simulink model "radarSim3"  (R2023b)
settings: Solver=VariableStepAuto  StartTime=0.0  StopTime=simTime  RelTol=1e-3
values from neighbouring files (symbols this model uses):
  c = get(groot,'defaultAxesColorOrder')    [compareData.m]
undefined symbols (not defined in the file or in its folder): fs, txDf_Dt, windowLen
libraries: dspsrcs4 x4, dspstat3 x2, dspxfrm3 x2
settings Model: Creator=pbroo  LastModifiedBy=pbroo

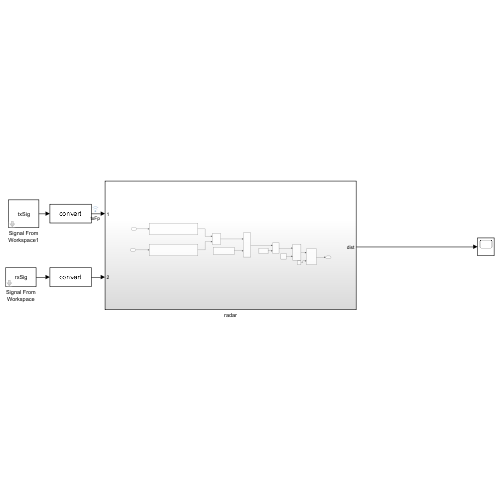
[thumbnail: Simulink's stored preview of the top-level diagram]
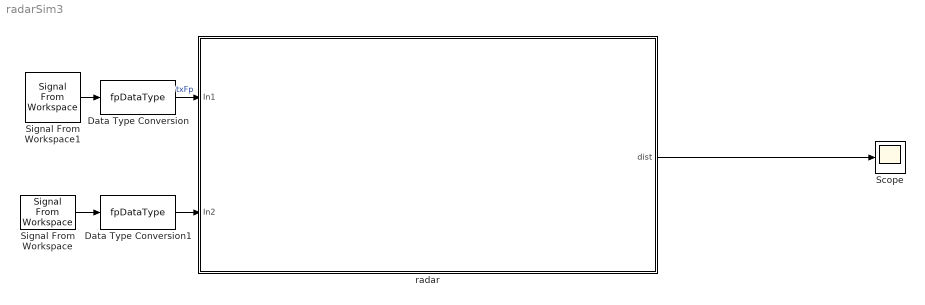
== system radarSim3 ==
  Data Type Conversion : DataTypeConversion  OutDataTypeStr=fpDataType  SaturateOnIntegerOverflow=off  RndMeth=Floor
  Data Type Conversion1 : DataTypeConversion  OutDataTypeStr=fpDataType  SaturateOnIntegerOverflow=off  RndMeth=Floor
  Scope : Scope
  Signal From Workspace : dspsrcs4/Signal From Workspace  X=rxSig  Ts=1  nsamps=1  OutputAfterFinalValue=Setting to zero  ignoreOrWarnInputAndFrameLengths=off  OutputFrames=off
  Signal From Workspace1 : dspsrcs4/Signal From Workspace  X=txSig  Ts=1  nsamps=1  OutputAfterFinalValue=Setting to zero  ignoreOrWarnInputAndFrameLengths=off  OutputFrames=off
  radar : Subsystem
  wires:
  Signal From Workspace1/1 -> Data Type Conversion/1
  Signal From Workspace/1 -> Data Type Conversion1/1
  radar/1(dist) -> Scope/1
  Data Type Conversion/1 -> radar/1(In1)  "txFp"
  Data Type Conversion1/1 -> radar/2(In2)

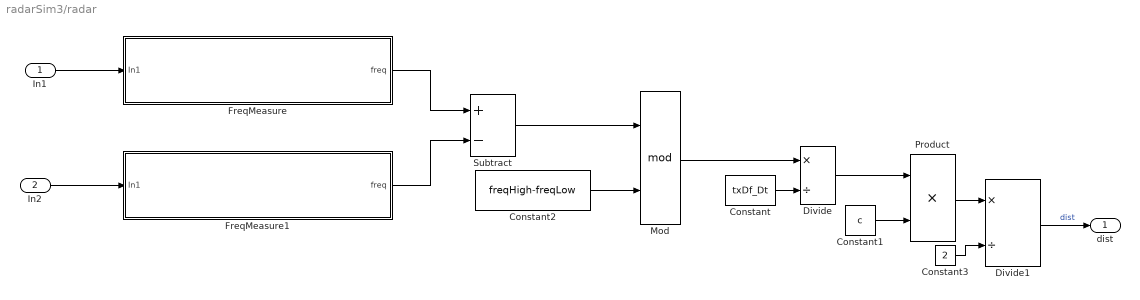
== system radarSim3/radar ==
  In1 : Inport
  In2 : Inport  Port=2
  Constant : Constant  Value=txDf_Dt
  Constant1 : Constant  Value=c
  Constant2 : Constant  Value=freqHigh-freqLow
  Constant3 : Constant  Value=2  VectorParams1D=off  SampleTime=-1
  Divide : Product  Inputs=*/
  Divide1 : Product  Inputs=*/
  FreqMeasure : Subsystem
  FreqMeasure1 : Subsystem
  Mod : Math  Operator=mod  SignedPower=on
  Product : Product
  Subtract : Sum  Inputs=+-
  dist : Outport
  wires:
  Subtract/1 -> Mod/1
  FreqMeasure1/1(freq) -> Subtract/2
  Constant/1 -> Divide/2
  Mod/1 -> Divide/1
  Divide/1 -> Product/1
  Constant1/1 -> Product/2
  FreqMeasure/1(freq) -> Subtract/1
  Constant2/1 -> Mod/2
  In1/1 -> FreqMeasure/1(In1)
  In2/1 -> FreqMeasure1/1(In1)
  Product/1 -> Divide1/1
  Divide1/1 -> dist/1  "dist"
  Constant3/1 -> Divide1/2

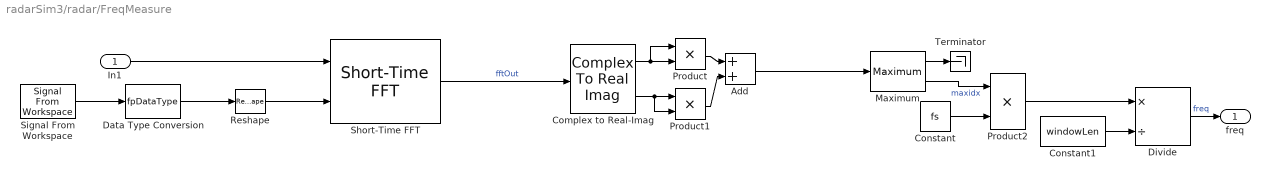
== system radarSim3/radar/FreqMeasure ==
  In1 : Inport
  Add : Sum
  Complex to Real-Imag : ComplexToRealImag
  Constant : Constant  Value=fs
  Constant1 : Constant  Value=windowLen
  Data Type Conversion : DataTypeConversion  OutDataTypeStr=fpDataType  SaturateOnIntegerOverflow=off  RndMeth=Floor
  Divide : Product  Inputs=*/
  Maximum : dspstat3/Maximum  operation=maximum  fcn=Value and Index  indexBase=One  operateOver=Each column  Dimension=1  InputProcessing=Columns as channels (frame based)  reset=None  roiEnable=off  roiType=Rectangles  roiPortion=Entire ROI  roiOutput=Individual statistics for each ROI  roiFlag=off  roundingMode=Floor  overflowMode=off  accumDataTypeStr=Inherit: Same as product output  accumLastDataTypeStr=Inherit: Same as product output
  Product : Product
  Product1 : Product
  Product2 : Product
  Reshape : Reshape  OutputDimensionality=Column vector (2-D)
  Short-Time FFT : dspxfrm3/Short-Time FFT  W=windowLen  OvLap=nOverlap  M=windowLen
  Signal From Workspace : dspsrcs4/Signal From Workspace  X=window  Ts=1  nsamps=1  OutputAfterFinalValue=Setting to zero  ignoreOrWarnInputAndFrameLengths=off  OutputFrames=off
  Terminator : Terminator
  freq : Outport
  wires:
  Maximum/2 -> Product2/1  "maxidx"
  Add/1 -> Maximum/1
  Constant1/1 -> Divide/2
  Constant/1 -> Product2/2
  Product2/1 -> Divide/1
  Divide/1 -> freq/1  "freq"
  Maximum/1 -> Terminator/1
  Short-Time FFT/1 -> Complex to Real-Imag/1  "fftOut"
  In1/1 -> Short-Time FFT/1
  Complex to Real-Imag/1 -> Product/1, Product/2
  Complex to Real-Imag/2 -> Product1/2, Product1/1
  Product/1 -> Add/1
  Product1/1 -> Add/2
  Signal From Workspace/1 -> Data Type Conversion/1
  Reshape/1 -> Short-Time FFT/2
  Data Type Conversion/1 -> Reshape/1

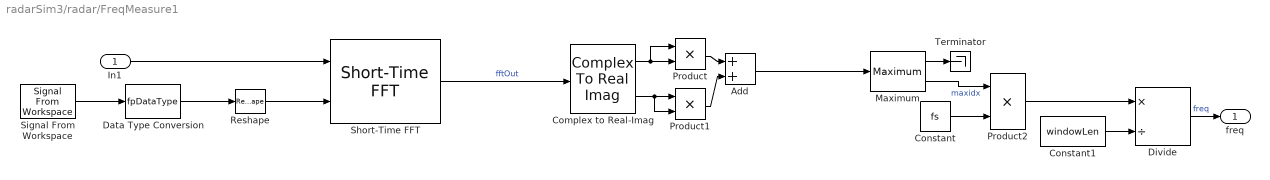
== system radarSim3/radar/FreqMeasure1 ==
  In1 : Inport
  Add : Sum
  Complex to Real-Imag : ComplexToRealImag
  Constant : Constant  Value=fs
  Constant1 : Constant  Value=windowLen
  Data Type Conversion : DataTypeConversion  OutDataTypeStr=fpDataType  SaturateOnIntegerOverflow=off  RndMeth=Floor
  Divide : Product  Inputs=*/
  Maximum : dspstat3/Maximum  operation=maximum  fcn=Value and Index  indexBase=One  operateOver=Each column  Dimension=1  InputProcessing=Columns as channels (frame based)  reset=None  roiEnable=off  roiType=Rectangles  roiPortion=Entire ROI  roiOutput=Individual statistics for each ROI  roiFlag=off  roundingMode=Floor  overflowMode=off  accumDataTypeStr=Inherit: Same as product output  accumLastDataTypeStr=Inherit: Same as product output
  Product : Product
  Product1 : Product
  Product2 : Product
  Reshape : Reshape  OutputDimensionality=Column vector (2-D)
  Short-Time FFT : dspxfrm3/Short-Time FFT  W=windowLen  OvLap=nOverlap  M=windowLen
  Signal From Workspace : dspsrcs4/Signal From Workspace  X=window  Ts=1  nsamps=1  OutputAfterFinalValue=Setting to zero  ignoreOrWarnInputAndFrameLengths=off  OutputFrames=off
  Terminator : Terminator
  freq : Outport
  wires:
  Maximum/2 -> Product2/1  "maxidx"
  Add/1 -> Maximum/1
  Constant1/1 -> Divide/2
  Constant/1 -> Product2/2
  Product2/1 -> Divide/1
  Divide/1 -> freq/1  "freq"
  Maximum/1 -> Terminator/1
  Short-Time FFT/1 -> Complex to Real-Imag/1  "fftOut"
  In1/1 -> Short-Time FFT/1
  Complex to Real-Imag/1 -> Product/1, Product/2
  Complex to Real-Imag/2 -> Product1/2, Product1/1
  Product/1 -> Add/1
  Product1/1 -> Add/2
  Signal From Workspace/1 -> Data Type Conversion/1
  Reshape/1 -> Short-Time FFT/2
  Data Type Conversion/1 -> Reshape/1
